simulink model "SlidingModeControl"  (R2024a)
settings: Solver=ode4  StartTime=0.0  StopTime=5  RelTol=1e-3
values from neighbouring files (symbols this model uses):
  a = 2    [SlidingModeControl_simulink_export.m]
  alpha = 1    [SlidingModeControl_simulink_export.m]
  amplitude = 3    [SlidingModeControl_simulink_export.m]
  g = 1    [SlidingModeControl_simulink_export.m]
  K = 5    [SlidingModeControl_simulink_export.m]
  t_final = 8    [SlidingModeControl_simulink_export.m]
  t_inicial = 3    [SlidingModeControl_simulink_export.m]
  y0 = [2;2]    [SlidingModeControl_simulink_export.m]
settings Model: Creator=Guilherme  LastModifiedBy=Guilherme

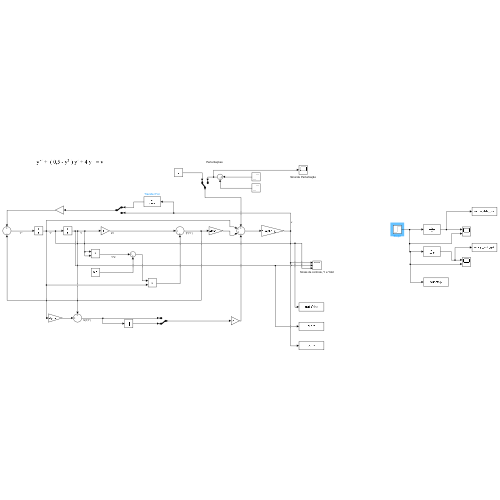
[thumbnail: Simulink's stored preview of the top-level diagram]
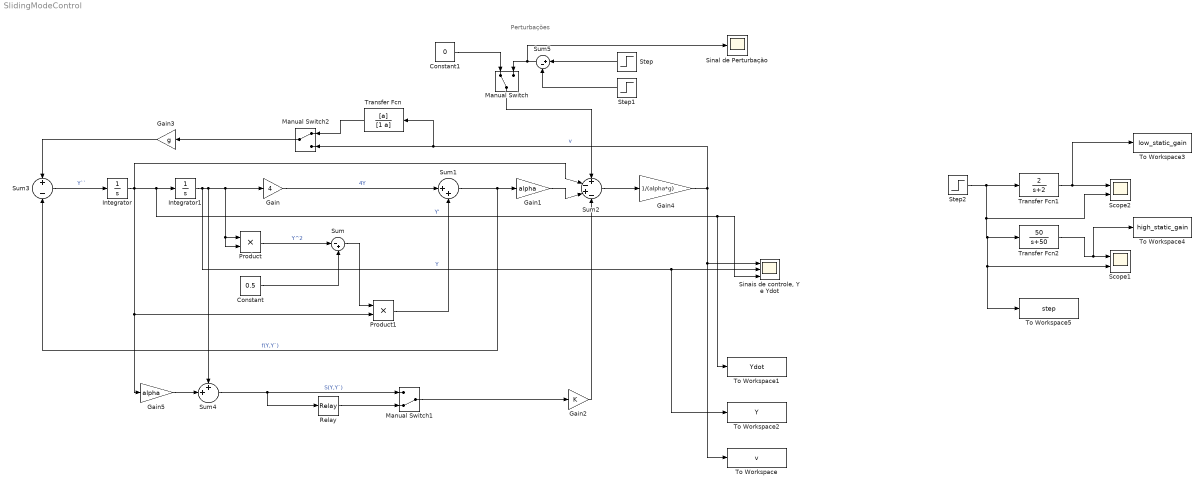
== system SlidingModeControl ==
  note: Perturbações
  Constant : Constant  Value=0.5
  Constant1 : Constant  Value=0
  Gain : Gain  Gain=4
  Gain1 : Gain  Gain=alpha
  Gain2 : Gain  Gain=K
  Gain3 : Gain  Gain=g
  Gain4 : Gain  Gain=1/(alpha*g)
  Gain5 : Gain  Gain=alpha
  Integrator : Integrator  InitialCondition=y0(2)
  Integrator1 : Integrator  InitialCondition=y0(1)
  Manual Switch : ManualSwitch
  Manual Switch1 : ManualSwitch  CurrentSetting=0
  Manual Switch2 : ManualSwitch
  Product : Product
  Product1 : Product
  Relay : Relay  OnSwitchValue=0  OffSwitchValue=0  OffOutputValue=-1
  Scope1 : Scope  NumInputPorts=2
  Scope2 : Scope  NumInputPorts=2
  "Sinais de controle, Y e Ydot" : Scope  NumInputPorts=3
  Sinal de Perturbação : Scope
  Step : Step  Time=t_inicial  After=amplitude  SampleTime=0
  Step1 : Step  Time=t_final  After=amplitude  SampleTime=0
  Step2 : Step  Time=0.000001  SampleTime=0
  Sum : Sum  Inputs=|-+
  Sum1 : Sum  Inputs=|++
  Sum2 : Sum  Inputs=+-+-
  Sum3 : Sum  Inputs=+|-
  Sum4 : Sum  Inputs=++|
  Sum5 : Sum  Inputs=|+-
  To Workspace : ToWorkspace  VariableName=v  SaveFormat=Timeseries  SampleTime=-1
  To Workspace1 : ToWorkspace  VariableName=Ydot  SaveFormat=Timeseries  SampleTime=-1
  To Workspace2 : ToWorkspace  VariableName=Y  SaveFormat=Timeseries  SampleTime=-1
  To Workspace3 : ToWorkspace  VariableName=low_static_gain  SaveFormat=Timeseries  SampleTime=-1
  To Workspace4 : ToWorkspace  VariableName=high_static_gain  SaveFormat=Timeseries  SampleTime=-1
  To Workspace5 : ToWorkspace  VariableName=step  SaveFormat=Timeseries  SampleTime=-1
  Transfer Fcn : TransferFcn  Numerator=[a]  Denominator=[1 a]
  Transfer Fcn1 : TransferFcn  Numerator=[2]  Denominator=[1 2]
  Transfer Fcn2 : TransferFcn  Numerator=[50]  Denominator=[1 50]
  wires:
  Integrator/1 -> Sum2/2, Gain5/1, Product1/2, To Workspace1/1, "Sinais de controle, Y e Ydot"/3, Integrator1/1  "Y'"
  Integrator1/1 -> To Workspace2/1, "Sinais de controle, Y e Ydot"/2, Product/2, Product/1, Gain/1, Sum4/1  "Y"
  Product/1 -> Sum/1  "Y^2"
  Constant/1 -> Sum/2
  Sum/1 -> Product1/1
  Product1/1 -> Sum1/2
  Gain/1 -> Sum1/1  "4Y"
  Sum1/1 -> Sum3/2, Gain1/1  "f(Y,Y`)"
  Sum3/1 -> Integrator/1  "Y``"
  Sum2/1 -> Gain4/1
  Gain2/1 -> Sum2/4
  Gain3/1 -> Sum3/1
  Gain4/1 -> Transfer Fcn/1, Manual Switch2/2, To Workspace/1, "Sinais de controle, Y e Ydot"/1  "v"
  Gain5/1 -> Sum4/2
  Constant1/1 -> Manual Switch/1
  Gain1/1 -> Sum2/3
  Manual Switch/1 -> Sum2/1
  Manual Switch1/1 -> Gain2/1
  Sum4/1 -> Relay/1, Manual Switch1/1  "S(Y,Y`)"
  Relay/1 -> Manual Switch1/2
  Sum5/1 -> Sinal de Perturbação/1, Manual Switch/2
  Step/1 -> Sum5/1
  Step1/1 -> Sum5/2
  Manual Switch2/1 -> Gain3/1
  Transfer Fcn/1 -> Manual Switch2/1
  Step2/1 -> Scope2/2, To Workspace5/1, Scope1/2, Transfer Fcn2/1, Transfer Fcn1/1
  Transfer Fcn1/1 -> To Workspace3/1, Scope2/1
  Transfer Fcn2/1 -> To Workspace4/1, Scope1/1
